simulink model "lab4Buligin"  (Simulink 5.0)
settings: Solver=ode45  StartTime=0.0  StopTime=10.0  RelTol=1e-3
settings Model: LastModifiedBy=Imed

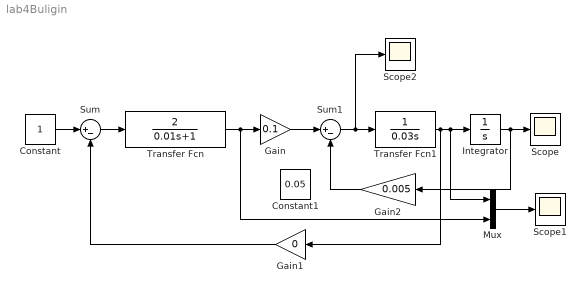
== system lab4Buligin ==
  Constant : Constant
  Constant1 : Constant  Value=0.05
  Gain : Gain  Gain=0.1  SaturateOnIntegerOverflow=on
  Gain1 : Gain  Orientation=left  Gain=0  SaturateOnIntegerOverflow=on
  Gain2 : Gain  Orientation=left  Gain=0.005  SaturateOnIntegerOverflow=on
  Integrator : Integrator
  Mux : Mux  Inputs=2
  Scope : Scope
      settings: TimeRange=10
  Scope1 : Scope
      settings: TimeRange=10  YMin=-2  YMax=12
  Scope2 : Scope
      settings: SaveName=ScopeData2
  Sum : Sum  Inputs=|+-  SaturateOnIntegerOverflow=on
  Sum1 : Sum  Inputs=|+-  SaturateOnIntegerOverflow=on
  Transfer Fcn : TransferFcn  Numerator=[2]  Denominator=[0.01 1]
  Transfer Fcn1 : TransferFcn  Denominator=[0.03 0]
  wires:
  Constant/1 -> Sum/1
  Sum/1 -> Transfer Fcn/1
  Gain/1 -> Sum1/1
  Integrator/1 -> Scope/1, Gain2/1
  Gain1/1 -> Sum/2
  Sum1/1 -> Transfer Fcn1/1, Scope2/1
  Transfer Fcn1/1 -> Gain1/1, Mux/1, Integrator/1
  Mux/1 -> Scope1/1
  Transfer Fcn/1 -> Gain/1, Mux/2
  Gain2/1 -> Sum1/2
